simulink model "RCseries1"  (R2020b)
settings: Solver=VariableStepAuto  StartTime=0.0  StopTime=10.0  RelTol=1e-3
values from neighbouring files (symbols this model uses):
  C = 1e-05    [data.mat]    (also in init.m)
  R = [10 5010 10010 15010 20010 25010]    [data.mat]    (also in init.m = R')
settings Model: Creator=vijay jagtap  LastModifiedBy=vijay jagtap

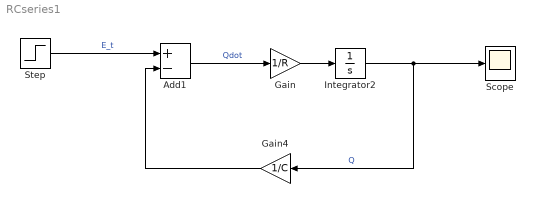
== system RCseries1 ==
  Add1 : Sum  Inputs=+-
  Gain : Gain  Gain=1/R
  Gain4 : Gain  Gain=1/C
  Integrator2 : Integrator
  Scope : Scope
  Step : Step  After=5  SampleTime=1
  wires:
  Step/1 -> Add1/1  "E_t"
  Add1/1 -> Gain/1  "Qdot"
  Integrator2/1 -> Gain4/1, Scope/1  "Q"
  Gain4/1 -> Add1/2
  Gain/1 -> Integrator2/1
